simulink model "model3"  (R2021b)
settings: Solver=ode23t  StartTime=0.0  StopTime=10  RelTol=1e-4
PreLoadFcn:
  | load('lookupTablesData.mat')
undefined symbols (not defined in the file): LUPTConv_inputCurrent, LUPTConv_Voutput, LUPTNewRep_outputCurrent, LUPTNewRep_Vinput, Temperature
libraries: spsCurrentMeasurementLib x5, spsDiodeLib x3, spsVoltageMeasurementLib x3, spsSeriesRLCBranchLib x2, spsControlledCurrentSourceLib x2, spsControlledVoltageSourceLib x2, spsDCVoltageSourceLib x1, spsGroundLib x1, spsIGBTDiodeLib x1, spsPWMGeneratorDCDCLib x1, spspowerguiLib x1
settings Model: ModifiedByFormat=DM  Creator=DM  LastModifiedBy=DM
settings SolverCC: AlgebraicLoopSolver=TrustRegion
settings DataIOCC: ReturnWorkspaceOutputs=off
settings DebuggingCC: SFMachineParentedDataDiag=warning  ArithmeticOperatorsInVariantConditions=warning
settings SFSimCC: SimUseLocalCustomCode=off  CustomCodeUndefinedFunction=UseInterfaceOnly
settings RTWCC: RTWUseLocalCustomCode=off
settings CodeAppCC: StateflowObjectComments=on
settings SimscapeCC: SimscapeNormalizeSystem=off

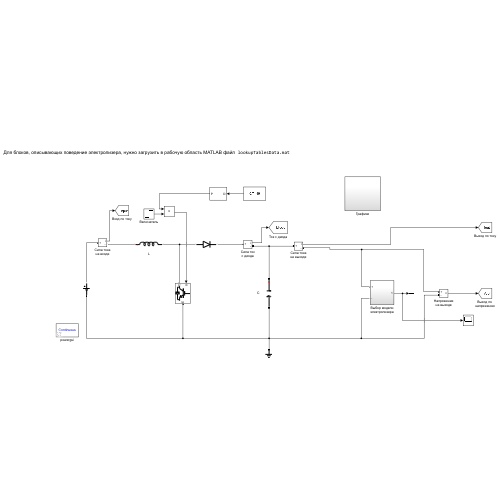
[thumbnail: Simulink's stored preview of the top-level diagram]
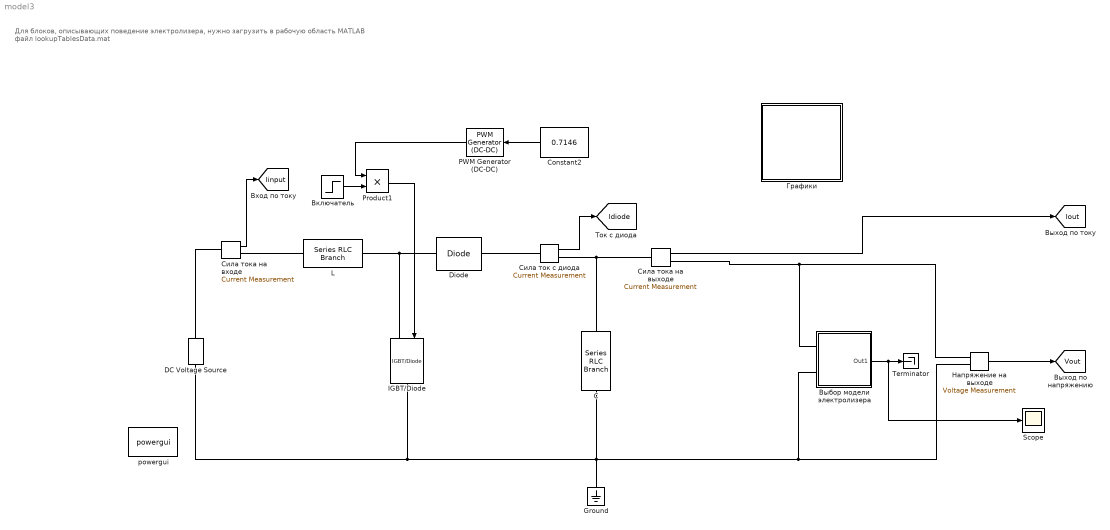
== system model3 ==
  note: Для блоков, описывающих поведение электролизера, нужно загрузить в рабочую область MATLAB файл lookupTablesData.mat
  "C " : spsSeriesRLCBranchLib/Series RLC Branch  LConnTagsString=__new0  RConnTagsString=__new0  BranchType=C  Resistance=1e-3  Inductance=1e-3  SetiL0=off  InitialCurrent=0  Capacitance=8000e-6  Setx0=off  InitialVoltage=40  Measurements=None
  Constant2 : Constant  Value=0.7146
  DC Voltage Source : spsDCVoltageSourceLib/DC Voltage Source  Amplitude=10  Measurements=None
  Diode : spsDiodeLib/Diode  Ron=0.001  Lon=0  Vf=0.1  IC=0  UseSnubber=off  Rs=inf  Cs=0  Measurements=off
  Ground : spsGroundLib/Ground  LConnTagsString=a
  IGBT/Diode : spsIGBTDiodeLib/IGBT//Diode  Ron=1e-3  Rs=1e5  Cs=inf  Measurements=off
  L : spsSeriesRLCBranchLib/Series RLC Branch  LConnTagsString=__new0  RConnTagsString=__new0  BranchType=L  Resistance=0.1  Inductance=0.001  SetiL0=off  InitialCurrent=0  Capacitance=1e-6  Setx0=off  InitialVoltage=0  Measurements=None
  PWM Generator (DC-DC) : spsPWMGeneratorDCDCLib/PWM Generator (DC-DC)  Fsw=10000  Ts=0
  Product1 : Product
  Scope : Scope
  Terminator : Terminator
  powergui : spspowerguiLib/powergui  Priority=1  SimulationMode=Continuous  SampleTime=0.1e-6  frequency=60  Iterations=50  frequencyindice=0  Pbase=100e6  ErrMax=1e-4  UnitsV=V  UnitsW=W  buscounter=0  FunctionMessages=off  echomessages=off  EnableUseOfTLC=off  CurrentSourceSwitches=on  DisableSnubberDevices=off  DisableRonSwitches=off  DisableVfSwitches=off  DisplayEquations=off  AutomaticDiscreteSolvers=off  SolverType=Tustin/Backward Euler (TBE)  Interpol=off  ExternalGateDelay=off  methode=off  Ts=10  x0status=zero  SPID=off  SwTol=0  HookPort=off  NonlinearTolerance=1e-4  nMaxIteration=100  ContinueOnMaxIteration=off  RestoreLinks=warning  ResistiveCurrentMeasurement=off  Frange=[0:2:500]  Ylog=off  Xlog=on  ShowGrid=off  save=off  variable=ZData  structure=0  ZoomFFT=off  StartTime=0.0  cycles=1  DisplayStyle=1  fundamental=60  FreqAxis=off  MaxFrequency=1000  frequencyindicesteady=1  RmsSteady=1  display=off
  Включатель : Step  Time=0.3  SampleTime=0
  Выбор модели электролизера : Subsystem
  Графики : Subsystem
  Напряжение на выходе : spsVoltageMeasurementLib/Voltage Measurement  PhasorSimulation=off  OutputType=Complex  PSBequivalent=0
  Сила ток с диода : spsCurrentMeasurementLib/Current Measurement  PhasorSimulation=off  OutputType=Complex  PSBequivalent=0
  Сила тока на входе : spsCurrentMeasurementLib/Current Measurement  PhasorSimulation=off  OutputType=Complex  PSBequivalent=0
  Сила тока на выходе : spsCurrentMeasurementLib/Current Measurement  PhasorSimulation=off  OutputType=Complex  PSBequivalent=0
  tag scope: Idiode=global, Iinput=global, Iout=global, Vout=global
  wires:
  Напряжение на выходе/1 -> [Vout]
  Сила тока на выходе/1 -> [Iout]
  Constant2/1 -> PWM Generator (DC-DC)/1
  Сила ток с диода/1 -> [Idiode]
  Сила тока на входе/1 -> [Iinput]
  Включатель/1 -> Product1/2
  Product1/1 -> IGBT/Diode/1
  PWM Generator (DC-DC)/1 -> Product1/1
  Выбор модели электролизера/1(Out1) -> Scope/1, Terminator/1
  connections:
  Напряжение на выходе/LConn2 -- Выбор модели электролизера/LConn2 -- Ground/LConn1 -- "C "/RConn1 -- DC Voltage Source/LConn1 -- IGBT/Diode/RConn1
  Напряжение на выходе/LConn1 -- Сила тока на выходе/RConn1 -- Выбор модели электролизера/LConn1
  Сила тока на выходе/LConn1 -- "C "/LConn1 -- Сила ток с диода/RConn1
  Сила тока на входе/LConn1 -- DC Voltage Source/RConn1
  Сила тока на входе/RConn1 -- L/LConn1
  L/RConn1 -- Diode/LConn1 -- IGBT/Diode/LConn1
  Diode/RConn1 -- Сила ток с диода/LConn1

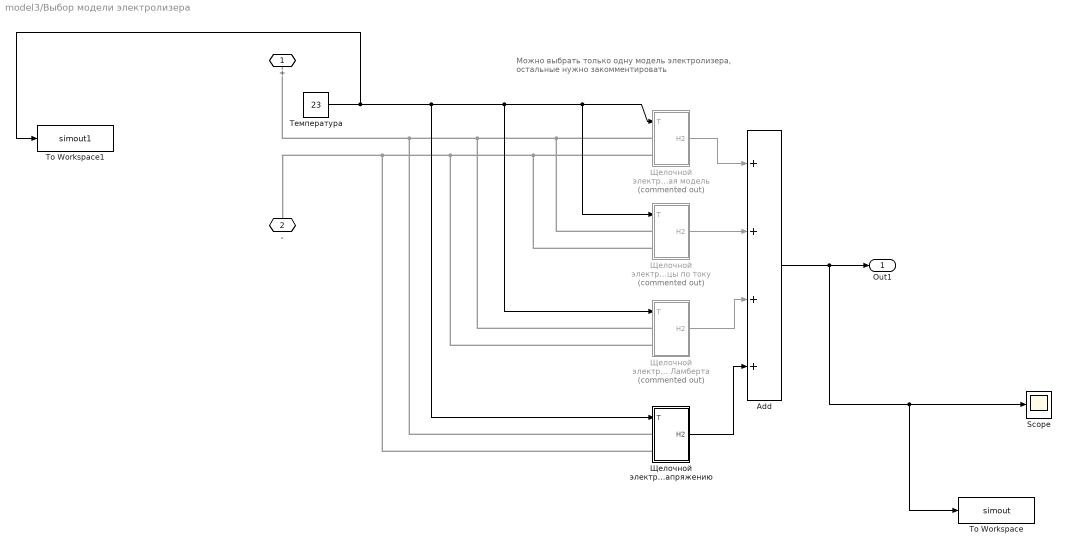
== system model3/Выбор модели электролизера ==
  note: Можно выбрать только одну модель электролизера,
      | остальные нужно закомментировать
  Add : Sum  Inputs=4
  Scope : Scope
  To Workspace : ToWorkspace  VariableName=simout  SaveFormat=Timeseries  SampleTime=-1
  To Workspace1 : ToWorkspace  VariableName=simout1  SaveFormat=Timeseries  SampleTime=-1
  Температура : Constant  Value=23
  Щелочной электролизер Поисковая таблица по напряжению : Subsystem  mask{A=0.25, nc=21}
      mask prompts: A "Area"; nc "Cells In series"
      mask help:
      | Базовая модель электролизера с поисковой таблицей по I-V кривым с использованием инвертированной эмпирической модели Уллеберга
      |
      | Молярный расход водорода определяется как
      | nH = ( f2(I/A)^2/(f1 + (I/A)^2 )(I/zF)
      | где:
      | f1, f2 - Пареаметры, связанные с эффективностью Фарадея
      | F - постоянная Фарадея = 96 485
      | z=2 - число электронов
      |
      | Положительные и отрицательные выводы элемента обозначаются знаками + и - соответственно.
  Щелочной электролизер Символьная функция Ламберта : Subsystem  Commented=on  mask{A=0.25, nc=21, r1=0.0001969, r2=-5.754e-07, s=0.1862, t1=0.008887, t2=-21.46, t3=2362}
      mask prompts: A "Area"; nc "Cells In series"; r1 "r1 ohmic parameter"; r2 "r2 ohmic parameter"; s "s overvoltage parameter"; t1 "t1 overvoltage parameter"; t2 "t2 overvoltage parameter"; t3 "t3 overvoltage parameter"
      mask help:
      | Basic alkaline electrolyzer model
      | Inverse of Ulleberg model with a current-voltage (I-V) relationship.
      | The current is given in terms of the voltage using lambert W function:
      |
      | W(10^(1/s*(Velec/Nc - Vrev))  *  Term1) / Term2 - Term3 = Ielec
      |
      | where:
      | Term1 = 10^( (r1 + r2*T) / (s*t1 + s*t2/T + s*t3/T^2)) * ln(10)*(r1 + r2*T) / (s*t1 + s*t2/T + s*t3/T^2)
      | Term2 = ln(10) * (1/(s*A))*(r1+r2*T)
      | Term3 = A/(t1 + t2/T + t3/T^2)
      | T=Temperature
      | A=Area
      | r1,r2 Parameters related to ohmic resistance of electrolyte.
      | s,t1,t2,t3 Coefficients for overvoltage on electrodes.
      | Vrev= 1.229
      |
      | Hydrogen molar flow rate is given by
      | nH = ( f2(I/A)^2/(f1 + (I/A)^2 )(I/zF)
      | where:
      | f1, f2 Pareameters related to the Faraday efficiency
      | F faraday constant = 96 485
      | z=2
      |
      |
      | The positive and negative terminals of the element are denoted by the + and - signs respectively.
  Щелочной электролизер Традиционная модель : Subsystem  Commented=on  mask{A=0.25, nc=21, r1=0.0001969, r2=-5.754e-07, s=0.1862, t1=0.008887, t2=-21.46, t3=2362}
      mask prompts: A "Area"; nc "Cells In series"; r1 "r1 ohmic parameter"; r2 "r2 ohmic parameter"; s "s overvoltage parameter"; t1 "t1 overvoltage parameter"; t2 "t2 overvoltage parameter"; t3 "t3 overvoltage parameter"
      mask help:
      | Basic alkaline electrolyzer model
      | The voltage-current (V-I) relationship for this element according to Ulleberg model is
      | V= Vrev + (r1+r2T)I/A + slog((t1+t2/T+t3/T^2)I/A+1)
      | where:
      | T=Temperature
      | A=Area
      | r1,r2 Parameters related to ohmic resistance of electrolyte.
      | s,t1,t2,t3 Coefficients for overvoltage on electrodes.
      | Vrev= 1.229
      |
      | Hydrogen molar flow rate is given by
      | nH = ( f2(I/A)^2/(f1 + (I/A)^2 )(I/zF)
      | where:
      | f1, f2 Pareameters related to the Faraday efficiency
      | F faraday constant = 96 485
      | z=2
      |
      |
      | The positive and negative terminals of the element are denoted by the + and - signs respectively.
  Щелочной электролизер Традиционная модель с использованием поисковой таблицы по току : Subsystem  Commented=on  mask{A=0.25, nc=21}
      mask prompts: A "Area"; nc "Cells In series"
      mask help:
      | Basic electrolyzer model - Lookup table for V-I curves using Ulleberg model
      |
      | Hydrogen molar flow rate is given by
      | nH = ( f2(I/A)^2/(f1 + (I/A)^2 )(I/zF)
      | where:
      | f1, f2 Pareameters related to the Faraday efficiency
      | F faraday constant = 96 485
      | z=2
      |
      | The positive and negative terminals of the element are denoted by the + and - signs respectively.
  + : PMIOPort  Side=Left
  - : PMIOPort  Port=2  Side=Left
  Out1 : Outport  VectorParamsAs1DForOutWhenUnconnected=off
  wires:
  Add/1 -> To Workspace/1, Scope/1, Out1/1
  Щелочной электролизер Традиционная модель с использованием поисковой таблицы по току/1(H2) -> Add/2
  Щелочной электролизер Символьная функция Ламберта/1(H2) -> Add/3
  Щелочной электролизер Традиционная модель/1(H2) -> Add/1
  Щелочной электролизер Поисковая таблица по напряжению/1(H2) -> Add/4
  Температура/1 -> To Workspace1/1, Щелочной электролизер Поисковая таблица по напряжению/1(T), Щелочной электролизер Символьная функция Ламберта/1(T), Щелочной электролизер Традиционная модель/1(T), Щелочной электролизер Традиционная модель с использованием поисковой таблицы по току/1(T)
  connections:
  Щелочной электролизер Традиционная модель с использованием поисковой таблицы по току/LConn2 -- Щелочной электролизер Поисковая таблица по напряжению/LConn2 -- -/RConn1 -- Щелочной электролизер Символьная функция Ламберта/LConn2 -- Щелочной электролизер Традиционная модель/LConn2
  Щелочной электролизер Традиционная модель с использованием поисковой таблицы по току/LConn1 -- Щелочной электролизер Поисковая таблица по напряжению/LConn1 -- +/RConn1 -- Щелочной электролизер Символьная функция Ламберта/LConn1 -- Щелочной электролизер Традиционная модель/LConn1

== system model3/Графики ==
  Scopes : Scope  NumInputPorts=4
  wires:
  [Iinput] -> Scopes/1
  [Vout] -> Scopes/3
  [Iout] -> Scopes/4
  [Idiode] -> Scopes/2

== system model3/Выбор модели электролизера/Щелочной электролизер Поисковая таблица по напряжению ==
  T : Inport
  Controlled Current Source : spsControlledCurrentSourceLib/Controlled Current Source  Initialize=on  Source_Type=DC  Amplitude=0  Phase=0  Frequency=0  Measurements=None
  Voltage Measurement : spsVoltageMeasurementLib/Voltage Measurement  PhasorSimulation=off  OutputType=Complex  PSBequivalent=0
  Модель электролизера : Subsystem  TreatAsAtomicUnit=on
  + : PMIOPort  Tag=PMCPort  Side=Left
  - : PMIOPort  Tag=PMCPort  Port=2  Side=Left
  H2 : Outport  VectorParamsAs1DForOutWhenUnconnected=off
  wires:
  Модель электролизера/2(M-h2) -> H2/1
  T/1 -> Модель электролизера/1(T)
  Модель электролизера/1(Ielec) -> Controlled Current Source/1
  Voltage Measurement/1 -> Модель электролизера/2(Velec)
  connections:
  -/RConn1 -- Controlled Current Source/RConn1 -- Voltage Measurement/LConn2
  Voltage Measurement/LConn1 -- +/RConn1 -- Controlled Current Source/LConn1

== system model3/Выбор модели электролизера/Щелочной электролизер Символьная функция Ламберта ==
  T : Inport
  Alkaline Electrolyzer Model : Subsystem  TreatAsAtomicUnit=on
  Controlled Current Source : spsControlledCurrentSourceLib/Controlled Current Source  Initialize=on  Source_Type=DC  Amplitude=0  Phase=0  Frequency=0  Measurements=None
  Voltage Measurement : spsVoltageMeasurementLib/Voltage Measurement  PhasorSimulation=off  OutputType=Complex  PSBequivalent=0
  + : PMIOPort  Tag=PMCPort  Side=Left
  - : PMIOPort  Tag=PMCPort  Port=2  Side=Left
  H2 : Outport  VectorParamsAs1DForOutWhenUnconnected=off
  wires:
  Alkaline Electrolyzer Model/2(M-h2) -> H2/1
  T/1 -> Alkaline Electrolyzer Model/1(T)
  Alkaline Electrolyzer Model/1(Ielec) -> Controlled Current Source/1
  Voltage Measurement/1 -> Alkaline Electrolyzer Model/2(Velec)
  connections:
  -/RConn1 -- Controlled Current Source/RConn1 -- Voltage Measurement/LConn2
  Voltage Measurement/LConn1 -- +/RConn1 -- Controlled Current Source/LConn1

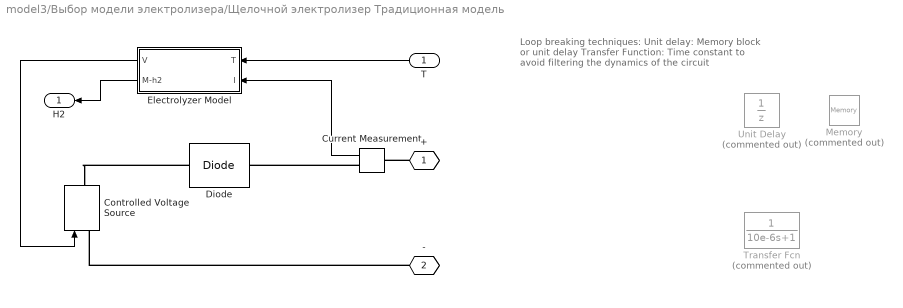
== system model3/Выбор модели электролизера/Щелочной электролизер Традиционная модель ==
  note: Loop breaking techniques:
      |
      | Unit delay: Memory block or unit delay
      |
      |
      |
      |
      |
      |
      |
      | Transfer Function: Time constant to avoid filtering
      | the dynamics of the circuit
  T : Inport
  Controlled Voltage Source : spsControlledVoltageSourceLib/Controlled Voltage Source  Initialize=on  Source_Type=DC  Amplitude=0  Phase=0  Frequency=0  Measurements=None
  Current Measurement : spsCurrentMeasurementLib/Current Measurement  PhasorSimulation=off  OutputType=Complex  PSBequivalent=0
  Diode : spsDiodeLib/Diode  Ron=0.00001  Lon=0  Vf=0.001  IC=0  UseSnubber=off  Rs=inf  Cs=0  Measurements=off
  Electrolyzer Model : Subsystem  TreatAsAtomicUnit=on
  Memory : Memory  Commented=on
  Transfer Fcn : TransferFcn  Commented=on  Denominator=[10e-6 1]
  Unit Delay : UnitDelay  Commented=on  SampleTime=-1  HasFrameUpgradeWarning=on
  + : PMIOPort  Tag=PMCPort  Side=Left
  - : PMIOPort  Tag=PMCPort  Port=2  Side=Left
  H2 : Outport  VectorParamsAs1DForOutWhenUnconnected=off
  wires:
  Electrolyzer Model/2(M-h2) -> H2/1
  T/1 -> Electrolyzer Model/1(T)
  Electrolyzer Model/1(V) -> Controlled Voltage Source/1
  Current Measurement/1 -> Electrolyzer Model/2(I)
  connections:
  -/RConn1 -- Controlled Voltage Source/LConn1
  +/RConn1 -- Current Measurement/LConn1
  Current Measurement/RConn1 -- Diode/LConn1
  Diode/RConn1 -- Controlled Voltage Source/RConn1

== system model3/Выбор модели электролизера/Щелочной электролизер Традиционная модель с использованием поисковой таблицы по току ==
  T : Inport
  Controlled Voltage Source : spsControlledVoltageSourceLib/Controlled Voltage Source  Initialize=on  Source_Type=DC  Amplitude=0  Phase=0  Frequency=0  Measurements=None
  Current Measurement : spsCurrentMeasurementLib/Current Measurement  PhasorSimulation=off  OutputType=Complex  PSBequivalent=0
  Diode : spsDiodeLib/Diode  Ron=0.00001  Lon=0  Vf=0.001  IC=0  UseSnubber=off  Rs=inf  Cs=0  Measurements=off
  Electrolyzer Model : Subsystem  TreatAsAtomicUnit=on
  + : PMIOPort  Tag=PMCPort  Side=Left
  - : PMIOPort  Tag=PMCPort  Port=2  Side=Left
  H2 : Outport  VectorParamsAs1DForOutWhenUnconnected=off
  wires:
  Electrolyzer Model/2(M-h2) -> H2/1
  T/1 -> Electrolyzer Model/1(T)
  Electrolyzer Model/1(Velec) -> Controlled Voltage Source/1
  Current Measurement/1 -> Electrolyzer Model/2(Ielec)
  connections:
  Current Measurement/LConn1 -- +/RConn1
  Current Measurement/RConn1 -- Diode/LConn1
  Diode/RConn1 -- Controlled Voltage Source/RConn1
  Controlled Voltage Source/LConn1 -- -/RConn1

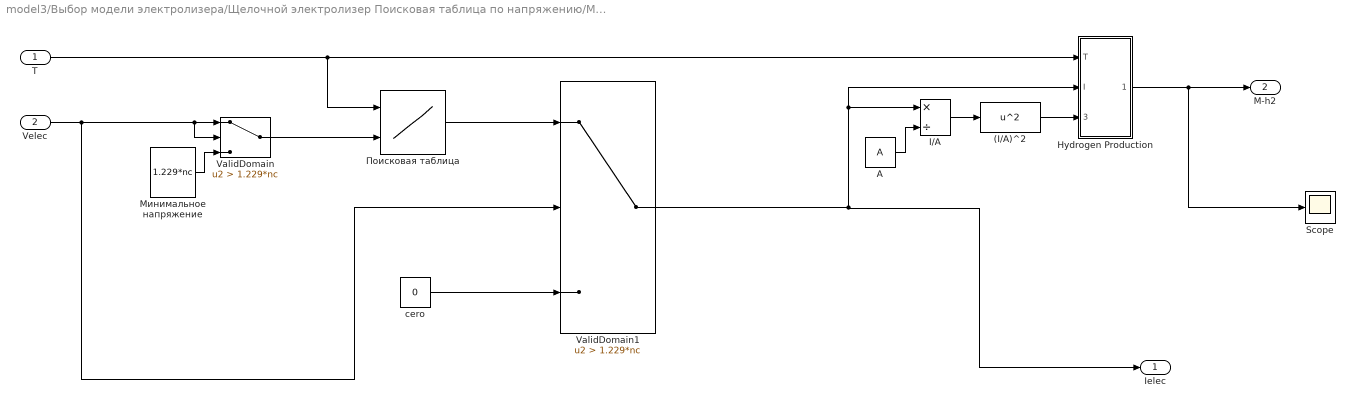
== system model3/Выбор модели электролизера/Щелочной электролизер Поисковая таблица по напряжению/Модель электролизера ==
  T : Inport
  Velec : Inport  Port=2
  (I/A)^2 : Fcn  Expr=u^2
  A : Constant  Value=A
  Hydrogen Production : Subsystem
  I/A : Product  Inputs=*/
  Scope : Scope
  ValidDomain : Switch  Criteria=u2 > Threshold  Threshold=1.229*nc
  ValidDomain1 : Switch  Criteria=u2 > Threshold  Threshold=1.229*nc
  cero : Constant  Value=0
  Минимальное напряжение : Constant  Value=1.229*nc
  Поисковая таблица : Lookup_n-D  BreakpointsForDimension1=Temperature  BreakpointsForDimension2=LUPTNewRep_Vinput  BreakpointsForDimension3=[5, 7]  BeginIndexSearchUsingPreviousIndexResult=on  Table=LUPTNewRep_outputCurrent  InternalRulePriority=Speed  RndMeth=Simplest  InputSameDT=on
      settings: InputPortMap=u0,u1
  Ielec : Outport  VectorParamsAs1DForOutWhenUnconnected=off
  M-h2 : Outport  Port=2  VectorParamsAs1DForOutWhenUnconnected=off
  wires:
  T/1 -> Поисковая таблица/1, Hydrogen Production/1(T)
  A/1 -> I/A/2
  I/A/1 -> (I/A)^2/1
  (I/A)^2/1 -> Hydrogen Production/3((I/A)^2)
  Hydrogen Production/1(mH2) -> Scope/1, M-h2/1
  Поисковая таблица/1 -> ValidDomain1/1
  ValidDomain1/1 -> Ielec/1, I/A/1, Hydrogen Production/2(I)
  Velec/1 -> ValidDomain/2, ValidDomain/1, ValidDomain1/2
  cero/1 -> ValidDomain1/3
  Минимальное напряжение/1 -> ValidDomain/3
  ValidDomain/1 -> Поисковая таблица/2

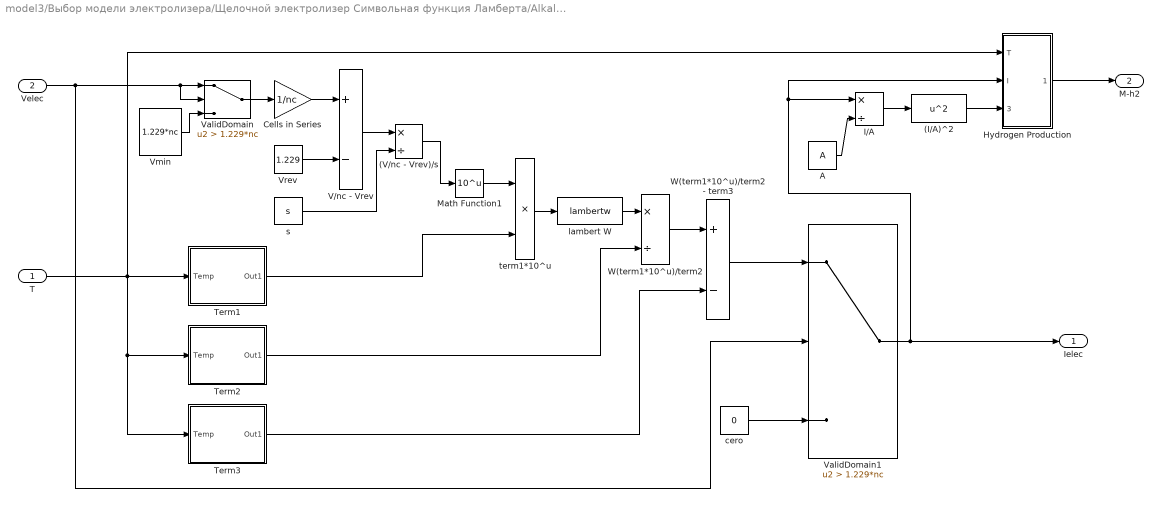
== system model3/Выбор модели электролизера/Щелочной электролизер Символьная функция Ламберта/Alkaline Electrolyzer Model ==
  T : Inport
  Velec : Inport  Port=2
  (I/A)^2 : Fcn  Expr=u^2
  (V/nc - Vrev)/s : Product  Inputs=*/
  A : Constant  Value=A
  Cells in Series : Gain  Gain=1/nc
  Hydrogen Production : Subsystem
  I/A : Product  Inputs=*/
  Math Function1 : Math  Operator=10^u  SignedPower=on  SaturateOnIntegerOverflow=on
  Term1 : Subsystem
  Term2 : Subsystem
  Term3 : Subsystem
  V/nc - Vrev : Sum  Inputs=+-
  ValidDomain : Switch  Criteria=u2 > Threshold  Threshold=1.229*nc
  ValidDomain1 : Switch  Criteria=u2 > Threshold  Threshold=1.229*nc
  Vmin : Constant  Value=1.229*nc
  Vrev : Constant  Value=1.229
  W(term1*10^u)/term2 : Product  Inputs=*/
  W(term1*10^u)/term2 - term3 : Sum  Inputs=+-
  cero : Constant  Value=0
  lambert W : MATLABFcn  MATLABFcn=lambertw
  s : Constant  Value=s
  term1*10^u : Product
  Ielec : Outport  VectorParamsAs1DForOutWhenUnconnected=off
  M-h2 : Outport  Port=2  VectorParamsAs1DForOutWhenUnconnected=off
  wires:
  T/1 -> Term3/1(Temp), Term2/1(Temp), Hydrogen Production/1(T), Term1/1(Temp)
  A/1 -> I/A/2
  I/A/1 -> (I/A)^2/1
  (I/A)^2/1 -> Hydrogen Production/3((I/A)^2)
  Hydrogen Production/1(mH2) -> M-h2/1
  term1*10^u/1 -> lambert W/1
  Cells in Series/1 -> V/nc - Vrev/1
  Vrev/1 -> V/nc - Vrev/2
  V/nc - Vrev/1 -> (V/nc - Vrev)/s/1
  s/1 -> (V/nc - Vrev)/s/2
  (V/nc - Vrev)/s/1 -> Math Function1/1
  Term1/1(Out1) -> term1*10^u/2
  Math Function1/1 -> term1*10^u/1
  lambert W/1 -> W(term1*10^u)/term2/1
  Term2/1(Out1) -> W(term1*10^u)/term2/2
  W(term1*10^u)/term2/1 -> W(term1*10^u)/term2 - term3/1
  Term3/1(Out1) -> W(term1*10^u)/term2 - term3/2
  ValidDomain/1 -> Cells in Series/1
  W(term1*10^u)/term2 - term3/1 -> ValidDomain1/1
  ValidDomain1/1 -> I/A/1, Hydrogen Production/2(I), Ielec/1
  Velec/1 -> ValidDomain/2, ValidDomain/1, ValidDomain1/2
  cero/1 -> ValidDomain1/3
  Vmin/1 -> ValidDomain/3

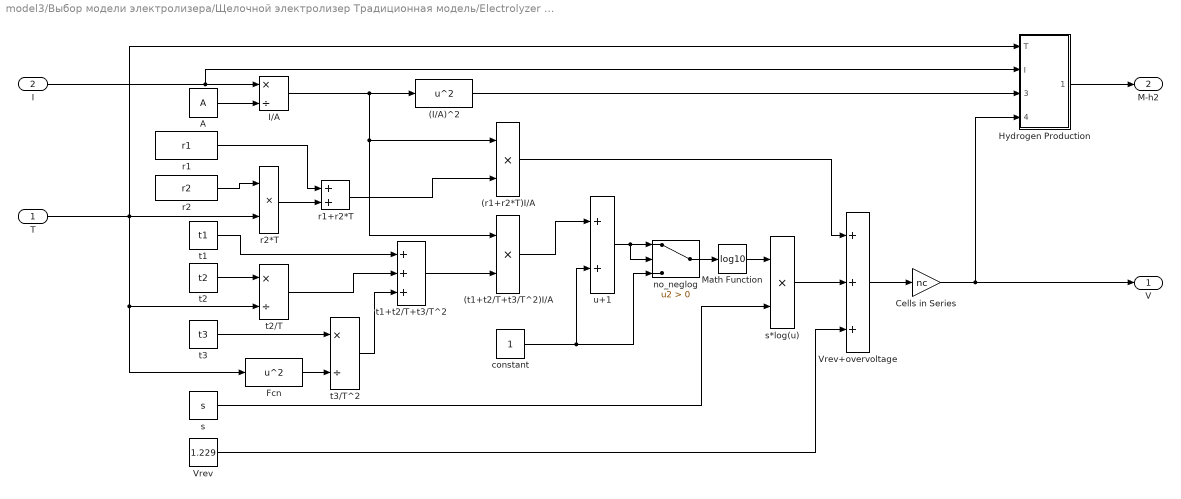
== system model3/Выбор модели электролизера/Щелочной электролизер Традиционная модель/Electrolyzer Model ==
  T : Inport
  I : Inport  Port=2
  (I/A)^2 : Fcn  Expr=u^2
  (r1+r2*T)I/A : Product
  (t1+t2/T+t3/T^2)I/A : Product
  A : Constant  Value=A
  Cells in Series : Gain  Gain=nc
  Fcn : Fcn  Expr=u^2
  Hydrogen Production : Subsystem
  I/A : Product  Inputs=*/
  Math Function : Math  Operator=log10  SignedPower=on  SaturateOnIntegerOverflow=on
  Vrev : Constant  Value=1.229
  Vrev+overvoltage : Sum  Inputs=+++
  constant : Constant
  no_neglog : Switch  Criteria=u2 > Threshold
  r1 : Constant  Value=r1
  r1+r2*T : Sum
  r2 : Constant  Value=r2
  r2*T : Product
  s : Constant  Value=s
  s*log(u) : Product
  t1 : Constant  Value=t1
  t1+t2/T+t3/T^2 : Sum  Inputs=+++
  t2 : Constant  Value=t2
  t2/T : Product  Inputs=*/
  t3 : Constant  Value=t3
  t3/T^2 : Product  Inputs=*/
  u+1 : Sum
  V : Outport  VectorParamsAs1DForOutWhenUnconnected=off
  M-h2 : Outport  Port=2  VectorParamsAs1DForOutWhenUnconnected=off
  wires:
  r2/1 -> r2*T/1
  r1/1 -> r1+r2*T/1
  r2*T/1 -> r1+r2*T/2
  I/1 -> Hydrogen Production/2(I), I/A/1
  t2/1 -> t2/T/1
  t3/1 -> t3/T^2/1
  Fcn/1 -> t3/T^2/2
  t1/1 -> t1+t2/T+t3/T^2/1
  t2/T/1 -> t1+t2/T+t3/T^2/2
  t3/T^2/1 -> t1+t2/T+t3/T^2/3
  T/1 -> Hydrogen Production/1(T), Fcn/1, t2/T/2, r2*T/2
  A/1 -> I/A/2
  I/A/1 -> (I/A)^2/1, (t1+t2/T+t3/T^2)I/A/1, (r1+r2*T)I/A/1
  r1+r2*T/1 -> (r1+r2*T)I/A/2
  t1+t2/T+t3/T^2/1 -> (t1+t2/T+t3/T^2)I/A/2
  constant/1 -> no_neglog/3, u+1/2
  s/1 -> s*log(u)/2
  Math Function/1 -> s*log(u)/1
  Vrev+overvoltage/1 -> Cells in Series/1
  (I/A)^2/1 -> Hydrogen Production/3((I/A)^2)
  Hydrogen Production/1(mH2) -> M-h2/1
  u+1/1 -> no_neglog/2, no_neglog/1
  no_neglog/1 -> Math Function/1
  (t1+t2/T+t3/T^2)I/A/1 -> u+1/1
  (r1+r2*T)I/A/1 -> Vrev+overvoltage/1
  s*log(u)/1 -> Vrev+overvoltage/2
  Vrev/1 -> Vrev+overvoltage/3
  Cells in Series/1 -> V/1, Hydrogen Production/4(Vcell)

== system model3/Выбор модели электролизера/Щелочной электролизер Традиционная модель с использованием поисковой таблицы по току/Electrolyzer Model ==
  T : Inport
  Ielec : Inport  Port=2
  (I/A)^2 : Fcn  Expr=u^2
  A : Constant  Value=A
  Hydrogen Production : Subsystem
  I/A : Product  Inputs=*/
  n-D Lookup Table : Lookup_n-D  BreakpointsForDimension1=Temperature  BreakpointsForDimension2=LUPTConv_inputCurrent  BreakpointsForDimension3=[5, 7]  BeginIndexSearchUsingPreviousIndexResult=on  Table=LUPTConv_Voutput  InternalRulePriority=Speed  RndMeth=Simplest  InputSameDT=on
      settings: InputPortMap=u0,u1
  Velec : Outport  VectorParamsAs1DForOutWhenUnconnected=off
  M-h2 : Outport  Port=2  VectorParamsAs1DForOutWhenUnconnected=off
  wires:
  T/1 -> Hydrogen Production/1(T), n-D Lookup Table/1
  Ielec/1 -> I/A/1, Hydrogen Production/2(I), n-D Lookup Table/2
  Hydrogen Production/1(mH2) -> M-h2/1
  (I/A)^2/1 -> Hydrogen Production/3((I/A)^2)
  A/1 -> I/A/2
  I/A/1 -> (I/A)^2/1
  n-D Lookup Table/1 -> Velec/1, Hydrogen Production/4(Vcell)

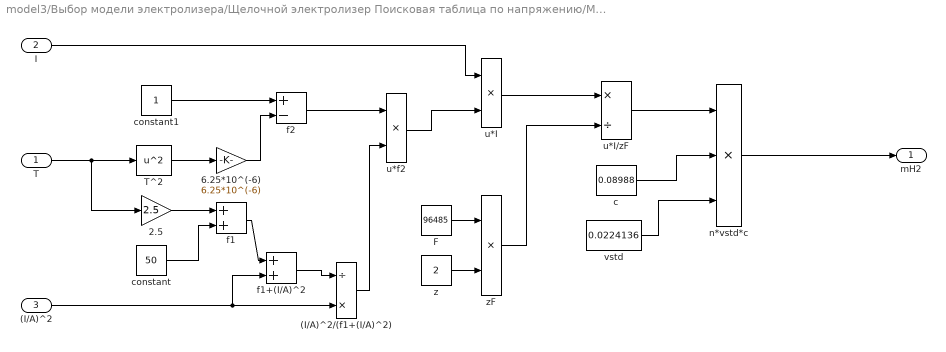
== system model3/Выбор модели электролизера/Щелочной электролизер Поисковая таблица по напряжению/Модель электролизера/Hydrogen Production ==
  T : Inport
  I : Inport  Port=2
  (I/A)^2 : Inport  Port=3
  (I/A)^2/(f1+(I/A)^2) : Product  Inputs=/*
  2.5 : Gain  Gain=2.5
  6.25*10^(-6) : Gain  Gain=6.25*10^(-6)
  F : Constant  Value=96485
  T^2 : Fcn  Expr=u^2
  c : Constant  Value=0.08988
  constant : Constant  Value=50
  constant1 : Constant
  f1 : Sum
  f1+(I/A)^2 : Sum
  f2 : Sum  Inputs=+-
  n*vstd*c : Product  Inputs=3
  u*I : Product
  u*I/zF : Product  Inputs=*/
  u*f2 : Product
  vstd : Constant  Value=0.0224136
  z : Constant  Value=2
  zF : Product
  mH2 : Outport  VectorParamsAs1DForOutWhenUnconnected=off
  wires:
  (I/A)^2/1 -> f1+(I/A)^2/2, (I/A)^2/(f1+(I/A)^2)/2
  constant/1 -> f1/2
  f1+(I/A)^2/1 -> (I/A)^2/(f1+(I/A)^2)/1
  (I/A)^2/(f1+(I/A)^2)/1 -> u*f2/2
  F/1 -> zF/1
  z/1 -> zF/2
  u*f2/1 -> u*I/2
  u*I/1 -> u*I/zF/1
  zF/1 -> u*I/zF/2
  u*I/zF/1 -> n*vstd*c/1
  c/1 -> n*vstd*c/2
  vstd/1 -> n*vstd*c/3
  2.5/1 -> f1/1
  f1/1 -> f1+(I/A)^2/1
  f2/1 -> u*f2/1
  constant1/1 -> f2/1
  T/1 -> 2.5/1, T^2/1
  T^2/1 -> 6.25*10^(-6)/1
  6.25*10^(-6)/1 -> f2/2
  n*vstd*c/1 -> mH2/1
  I/1 -> u*I/1

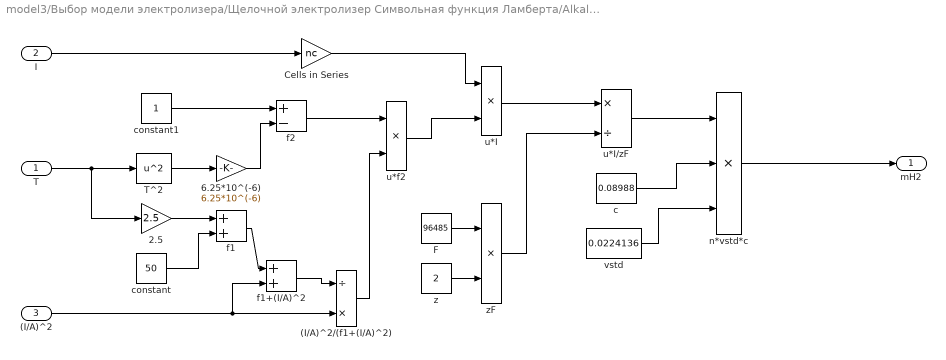
== system model3/Выбор модели электролизера/Щелочной электролизер Символьная функция Ламберта/Alkaline Electrolyzer Model/Hydrogen Production ==
  T : Inport
  I : Inport  Port=2
  (I/A)^2 : Inport  Port=3
  (I/A)^2/(f1+(I/A)^2) : Product  Inputs=/*
  2.5 : Gain  Gain=2.5
  6.25*10^(-6) : Gain  Gain=6.25*10^(-6)
  Cells in Series : Gain  Gain=nc
  F : Constant  Value=96485
  T^2 : Fcn  Expr=u^2
  c : Constant  Value=0.08988
  constant : Constant  Value=50
  constant1 : Constant
  f1 : Sum
  f1+(I/A)^2 : Sum
  f2 : Sum  Inputs=+-
  n*vstd*c : Product  Inputs=3
  u*I : Product
  u*I/zF : Product  Inputs=*/
  u*f2 : Product
  vstd : Constant  Value=0.0224136
  z : Constant  Value=2
  zF : Product
  mH2 : Outport  VectorParamsAs1DForOutWhenUnconnected=off
  wires:
  (I/A)^2/1 -> f1+(I/A)^2/2, (I/A)^2/(f1+(I/A)^2)/2
  constant/1 -> f1/2
  f1+(I/A)^2/1 -> (I/A)^2/(f1+(I/A)^2)/1
  (I/A)^2/(f1+(I/A)^2)/1 -> u*f2/2
  F/1 -> zF/1
  z/1 -> zF/2
  u*f2/1 -> u*I/2
  u*I/1 -> u*I/zF/1
  zF/1 -> u*I/zF/2
  u*I/zF/1 -> n*vstd*c/1
  c/1 -> n*vstd*c/2
  vstd/1 -> n*vstd*c/3
  I/1 -> Cells in Series/1
  2.5/1 -> f1/1
  f1/1 -> f1+(I/A)^2/1
  f2/1 -> u*f2/1
  constant1/1 -> f2/1
  T/1 -> 2.5/1, T^2/1
  T^2/1 -> 6.25*10^(-6)/1
  6.25*10^(-6)/1 -> f2/2
  n*vstd*c/1 -> mH2/1
  Cells in Series/1 -> u*I/1

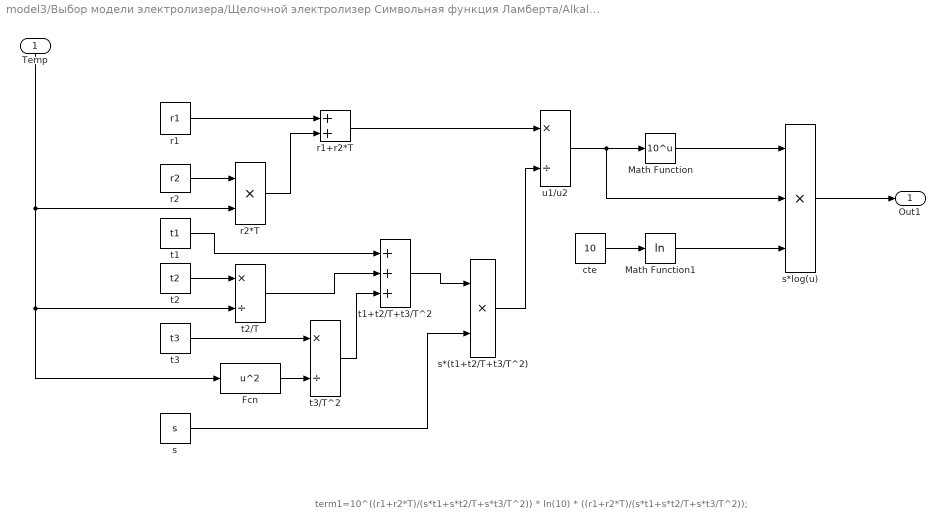
== system model3/Выбор модели электролизера/Щелочной электролизер Символьная функция Ламберта/Alkaline Electrolyzer Model/Term1 ==
  note: term1=10^((r1+r2*T)/(s*t1+s*t2/T+s*t3/T^2)) * ln(10) * ((r1+r2*T)/(s*t1+s*t2/T+s*t3/T^2));
  Temp : Inport
  Fcn : Fcn  Expr=u^2
  Math Function : Math  Operator=10^u  SignedPower=on  SaturateOnIntegerOverflow=on
  Math Function1 : Math  Operator=log  SignedPower=on  SaturateOnIntegerOverflow=on
  cte : Constant  Value=10
  r1 : Constant  Value=r1
  r1+r2*T : Sum
  r2 : Constant  Value=r2
  r2*T : Product
  s : Constant  Value=s
  s*(t1+t2/T+t3/T^2) : Product
  s*log(u) : Product  Inputs=3
  t1 : Constant  Value=t1
  t1+t2/T+t3/T^2 : Sum  Inputs=+++
  t2 : Constant  Value=t2
  t2/T : Product  Inputs=*/
  t3 : Constant  Value=t3
  t3/T^2 : Product  Inputs=*/
  u1/u2 : Product  Inputs=*/
  Out1 : Outport  VectorParamsAs1DForOutWhenUnconnected=off
  wires:
  t2/1 -> t2/T/1
  Fcn/1 -> t3/T^2/2
  t3/1 -> t3/T^2/1
  t1/1 -> t1+t2/T+t3/T^2/1
  t2/T/1 -> t1+t2/T+t3/T^2/2
  t3/T^2/1 -> t1+t2/T+t3/T^2/3
  r2/1 -> r2*T/1
  r1/1 -> r1+r2*T/1
  r2*T/1 -> r1+r2*T/2
  Temp/1 -> t2/T/2, Fcn/1, r2*T/2
  t1+t2/T+t3/T^2/1 -> s*(t1+t2/T+t3/T^2)/1
  s/1 -> s*(t1+t2/T+t3/T^2)/2
  r1+r2*T/1 -> u1/u2/1
  s*(t1+t2/T+t3/T^2)/1 -> u1/u2/2
  u1/u2/1 -> s*log(u)/2, Math Function/1
  Math Function/1 -> s*log(u)/1
  Math Function1/1 -> s*log(u)/3
  cte/1 -> Math Function1/1
  s*log(u)/1 -> Out1/1

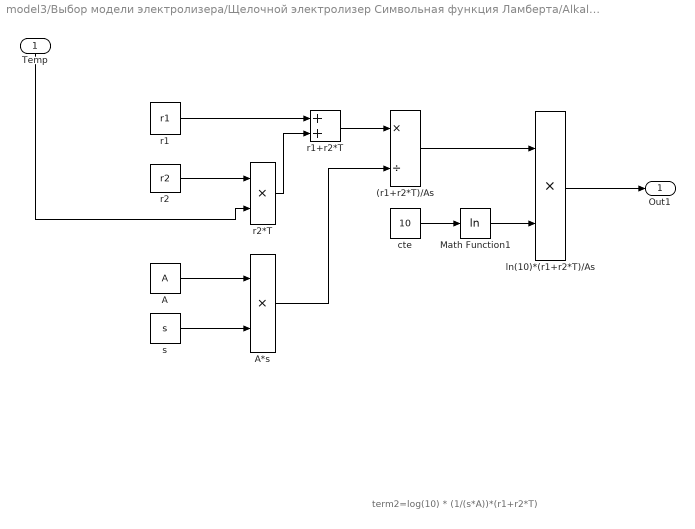
== system model3/Выбор модели электролизера/Щелочной электролизер Символьная функция Ламберта/Alkaline Electrolyzer Model/Term2 ==
  note: term2=log(10) * (1/(s*A))*(r1+r2*T)
  Temp : Inport
  (r1+r2*T)/As : Product  Inputs=*/
  A : Constant  Value=A
  A*s : Product
  Math Function1 : Math  Operator=log  SignedPower=on  SaturateOnIntegerOverflow=on
  cte : Constant  Value=10
  ln(10)*(r1+r2*T)/As : Product
  r1 : Constant  Value=r1
  r1+r2*T : Sum
  r2 : Constant  Value=r2
  r2*T : Product
  s : Constant  Value=s
  Out1 : Outport  VectorParamsAs1DForOutWhenUnconnected=off
  wires:
  r2/1 -> r2*T/1
  r1/1 -> r1+r2*T/1
  r2*T/1 -> r1+r2*T/2
  Temp/1 -> r2*T/2
  s/1 -> A*s/2
  r1+r2*T/1 -> (r1+r2*T)/As/1
  A*s/1 -> (r1+r2*T)/As/2
  (r1+r2*T)/As/1 -> ln(10)*(r1+r2*T)/As/1
  Math Function1/1 -> ln(10)*(r1+r2*T)/As/2
  cte/1 -> Math Function1/1
  ln(10)*(r1+r2*T)/As/1 -> Out1/1
  A/1 -> A*s/1

== system model3/Выбор модели электролизера/Щелочной электролизер Символьная функция Ламберта/Alkaline Electrolyzer Model/Term3 ==
  note: term3=A/(t1+t2/T+t3/T^2);
  Temp : Inport
  A : Constant  Value=A
  A/(t1+t2/T+t3/T^2) : Product  Inputs=*/
  Fcn : Fcn  Expr=u^2
  t1 : Constant  Value=t1
  t1+t2/T+t3/T^2 : Sum  Inputs=+++
  t2 : Constant  Value=t2
  t2/T : Product  Inputs=*/
  t3 : Constant  Value=t3
  t3/T^2 : Product  Inputs=*/
  Out1 : Outport  VectorParamsAs1DForOutWhenUnconnected=off
  wires:
  t2/1 -> t2/T/1
  Fcn/1 -> t3/T^2/2
  t3/1 -> t3/T^2/1
  t1/1 -> t1+t2/T+t3/T^2/1
  t2/T/1 -> t1+t2/T+t3/T^2/2
  t3/T^2/1 -> t1+t2/T+t3/T^2/3
  Temp/1 -> t2/T/2, Fcn/1
  t1+t2/T+t3/T^2/1 -> A/(t1+t2/T+t3/T^2)/2
  A/(t1+t2/T+t3/T^2)/1 -> Out1/1
  A/1 -> A/(t1+t2/T+t3/T^2)/1

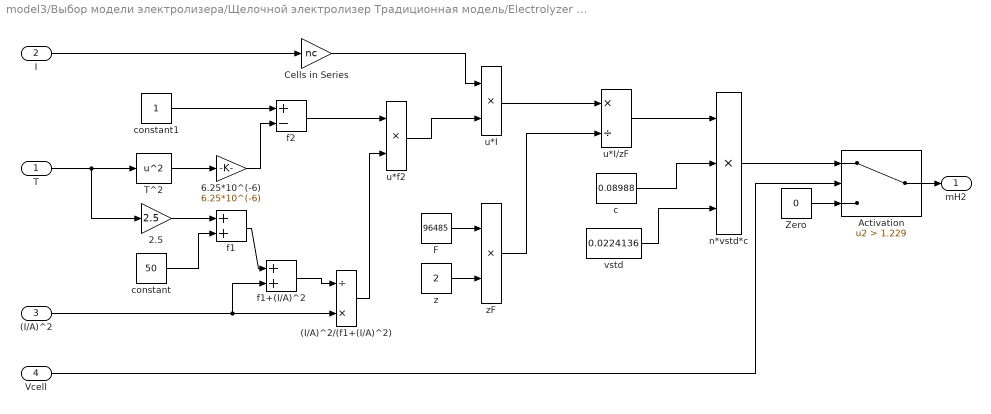
== system model3/Выбор модели электролизера/Щелочной электролизер Традиционная модель/Electrolyzer Model/Hydrogen Production ==
  T : Inport
  I : Inport  Port=2
  (I/A)^2 : Inport  Port=3
  Vcell : Inport  Port=4
  (I/A)^2/(f1+(I/A)^2) : Product  Inputs=/*
  2.5 : Gain  Gain=2.5
  6.25*10^(-6) : Gain  Gain=6.25*10^(-6)
  Activation : Switch  Criteria=u2 > Threshold  Threshold=1.229
  Cells in Series : Gain  Gain=nc
  F : Constant  Value=96485
  T^2 : Fcn  Expr=u^2
  Zero : Constant  Value=0
  c : Constant  Value=0.08988
  constant : Constant  Value=50
  constant1 : Constant
  f1 : Sum
  f1+(I/A)^2 : Sum
  f2 : Sum  Inputs=+-
  n*vstd*c : Product  Inputs=3
  u*I : Product
  u*I/zF : Product  Inputs=*/
  u*f2 : Product
  vstd : Constant  Value=0.0224136
  z : Constant  Value=2
  zF : Product
  mH2 : Outport  VectorParamsAs1DForOutWhenUnconnected=off
  wires:
  (I/A)^2/1 -> f1+(I/A)^2/2, (I/A)^2/(f1+(I/A)^2)/2
  constant/1 -> f1/2
  f1+(I/A)^2/1 -> (I/A)^2/(f1+(I/A)^2)/1
  (I/A)^2/(f1+(I/A)^2)/1 -> u*f2/2
  F/1 -> zF/1
  z/1 -> zF/2
  u*f2/1 -> u*I/2
  u*I/1 -> u*I/zF/1
  zF/1 -> u*I/zF/2
  u*I/zF/1 -> n*vstd*c/1
  c/1 -> n*vstd*c/2
  vstd/1 -> n*vstd*c/3
  I/1 -> Cells in Series/1
  2.5/1 -> f1/1
  f1/1 -> f1+(I/A)^2/1
  f2/1 -> u*f2/1
  constant1/1 -> f2/1
  T/1 -> 2.5/1, T^2/1
  T^2/1 -> 6.25*10^(-6)/1
  6.25*10^(-6)/1 -> f2/2
  n*vstd*c/1 -> Activation/1
  Vcell/1 -> Activation/2
  Activation/1 -> mH2/1
  Zero/1 -> Activation/3
  Cells in Series/1 -> u*I/1

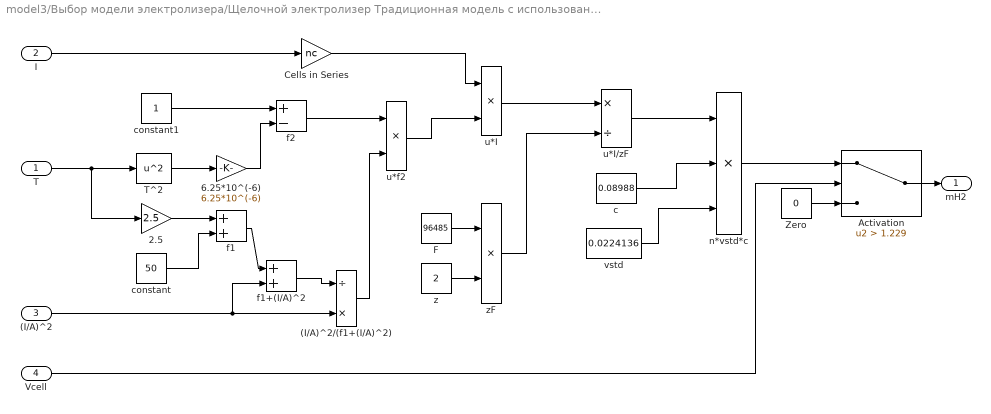
== system model3/Выбор модели электролизера/Щелочной электролизер Традиционная модель с использованием поисковой таблицы по току/Electrolyzer Model/Hydrogen Production ==
  T : Inport
  I : Inport  Port=2
  (I/A)^2 : Inport  Port=3
  Vcell : Inport  Port=4
  (I/A)^2/(f1+(I/A)^2) : Product  Inputs=/*
  2.5 : Gain  Gain=2.5
  6.25*10^(-6) : Gain  Gain=6.25*10^(-6)
  Activation : Switch  Criteria=u2 > Threshold  Threshold=1.229
  Cells in Series : Gain  Gain=nc
  F : Constant  Value=96485
  T^2 : Fcn  Expr=u^2
  Zero : Constant  Value=0
  c : Constant  Value=0.08988
  constant : Constant  Value=50
  constant1 : Constant
  f1 : Sum
  f1+(I/A)^2 : Sum
  f2 : Sum  Inputs=+-
  n*vstd*c : Product  Inputs=3
  u*I : Product
  u*I/zF : Product  Inputs=*/
  u*f2 : Product
  vstd : Constant  Value=0.0224136
  z : Constant  Value=2
  zF : Product
  mH2 : Outport  VectorParamsAs1DForOutWhenUnconnected=off
  wires:
  (I/A)^2/1 -> f1+(I/A)^2/2, (I/A)^2/(f1+(I/A)^2)/2
  constant/1 -> f1/2
  f1+(I/A)^2/1 -> (I/A)^2/(f1+(I/A)^2)/1
  (I/A)^2/(f1+(I/A)^2)/1 -> u*f2/2
  F/1 -> zF/1
  z/1 -> zF/2
  u*f2/1 -> u*I/2
  u*I/1 -> u*I/zF/1
  zF/1 -> u*I/zF/2
  u*I/zF/1 -> n*vstd*c/1
  c/1 -> n*vstd*c/2
  vstd/1 -> n*vstd*c/3
  I/1 -> Cells in Series/1
  2.5/1 -> f1/1
  f1/1 -> f1+(I/A)^2/1
  f2/1 -> u*f2/1
  constant1/1 -> f2/1
  T/1 -> 2.5/1, T^2/1
  T^2/1 -> 6.25*10^(-6)/1
  6.25*10^(-6)/1 -> f2/2
  n*vstd*c/1 -> Activation/1
  Vcell/1 -> Activation/2
  Activation/1 -> mH2/1
  Zero/1 -> Activation/3
  Cells in Series/1 -> u*I/1
